simulink model "HIL_Testing_SW"  (Simulink 7.5)
settings: Solver=ode1  StartTime=0.0  StopTime=Inf  FixedStep=0.001  RelTol=1e-3
PostLoadFcn:
  | , if any(exist('dsrtsu_mdlpostloadfcn', 'file') == [2, 3, 6]), try dsrtsu_mdlpostloadfcn('Execute', bdroot); catch fprintf('Error in PostLoadFcn (dsrtsu_mdlpostloadfcn) for model "%s":\n %s\n', bdroot, lasterr); end, end,
undefined symbols (not defined in the file): CeBSER_Cnt_NumTempAxisPts, ChargeCord, ChargeCord_Control, ChargeToSOCCurr, ChrgCurrLim, CrntSens1Fine, CS_SOCSetPt, CyclerMaxChrgPwr, CyclerMaxDschrgPwr, deltaAhr, Drive_1, Drive_10, Drive_11, Drive_12, Drive_13, Drive_14, Drive_15, Drive_16, Drive_17, Drive_18, Drive_19, Drive_2, Drive_20, Drive_21, Drive_22, Drive_23, Drive_24, Drive_25, Drive_26, Drive_27, Drive_28, Drive_29, Drive_3, Drive_30, Drive_31, Drive_32, Drive_33, Drive_34, Drive_35, Drive_36, Drive_37, Drive_38, Drive_39, Drive_4, Drive_40, Drive_41, Drive_42, Drive_43, Drive_44, Drive_45, Drive_46, Drive_47, Drive_48, Drive_49, Drive_5, Drive_50, Drive_51, Drive_6, Drive_7, Drive_8 ... (+50)
libraries: simulink x129, rtican x50, rti2211sailib x5, rti2211serlib x5, rti2202miolib x3
(part 7 of 23)

== system HIL_Testing_SW/LionsHeart/FeaturePresentation/Down_to_Business ==
  CyclerCurrent : Inport  OutDataType=fixdt(1, 16)  OutScaling=2^0
  CyclerVoltage : Inport  Port=2  OutDataType=fixdt(1, 16)  OutScaling=2^0
  BatTemp : Inport  Port=3  OutDataType=fixdt(1, 16)  OutScaling=2^0
  PackVoltage : Inport  Port=4  OutDataType=fixdt(1, 16)  OutScaling=2^0
  PackCurrent : Inport  Port=5  OutDataType=fixdt(1, 16)  OutScaling=2^0
  PackVolt_MaxCell : Inport  Port=6  OutDataType=fixdt(1, 16)  OutScaling=2^0
  PackVolt_MinCell : Inport  Port=7  OutDataType=fixdt(1, 16)  OutScaling=2^0
  Indicator : Inport  Port=8  OutDataType=fixdt(1, 16)  OutScaling=2^0
  CS_SwitchMode : Inport  Port=9  OutDataType=fixdt(1, 16)  OutScaling=2^0
  ESTOP : Inport  Port=10  OutDataType=fixdt(1, 16)  OutScaling=2^0
  ChrgCurrSelect_F : Inport  Port=11  OutDataType=fixdt(1, 16)  OutScaling=2^0
  SOC : Inport  Port=12  OutDataType=fixdt(1, 16)  OutScaling=2^0
  PwrCycle : Inport  Port=13  OutDataType=fixdt(1, 16)  OutScaling=2^0
  Voltage_Cntrl : Inport  Port=14  OutDataType=fixdt(1, 16)  OutScaling=2^0
  Current_Cntrl : Inport  Port=15  OutDataType=fixdt(1, 16)  OutScaling=2^0
  DriveProfile_ModeControl : Subsystem
  Profile_Data : Outport  OutDataType=fixdt(1, 16)  OutScaling=2^0
  CM : Outport  Port=2  OutDataType=fixdt(1, 16)  OutScaling=2^0
  ResetSOC : Outport  Port=3  OutDataType=fixdt(1, 16)  OutScaling=2^0
  VoltTarget : Outport  Port=4  OutDataType=fixdt(1, 16)  OutScaling=2^0
  IndicatorSF : Outport  Port=5  OutDataType=fixdt(1, 16)  OutScaling=2^0
  Profile_Mode : Outport  Port=6  OutDataType=fixdt(1, 16)  OutScaling=2^0
  Script_PwrCycle : Outport  Port=7  OutDataType=fixdt(1, 16)  OutScaling=2^0
  ChargeCurrSelect : Outport  Port=8  OutDataType=fixdt(1, 16)  OutScaling=2^0
  SetChamberT_ToBatTemp : Outport  Port=9  OutDataType=fixdt(1, 16)  OutScaling=2^0
  wires:
  CyclerCurrent/1 -> DriveProfile_ModeControl/1(Current)
  CyclerVoltage/1 -> DriveProfile_ModeControl/2(Voltage)
  BatTemp/1 -> DriveProfile_ModeControl/3(Temp)
  PackVoltage/1 -> DriveProfile_ModeControl/4(PackVoltage)
  PackVolt_MaxCell/1 -> DriveProfile_ModeControl/6(PackVolt_MaxCell)
  PackCurrent/1 -> DriveProfile_ModeControl/5(PackCurrent)
  PackVolt_MinCell/1 -> DriveProfile_ModeControl/7(PackVolt_MinCell)
  Indicator/1 -> DriveProfile_ModeControl/8(Indicator)
  CS_SwitchMode/1 -> DriveProfile_ModeControl/9(CS_ModeSwitch)
  DriveProfile_ModeControl/1(Profile_Data) -> Profile_Data/1
  DriveProfile_ModeControl/2(CM) -> CM/1
  DriveProfile_ModeControl/3(ResetSOC) -> ResetSOC/1
  DriveProfile_ModeControl/4(VoltTarget) -> VoltTarget/1
  DriveProfile_ModeControl/5(IndicatorSF) -> IndicatorSF/1
  DriveProfile_ModeControl/6(Profile_Mode) -> Profile_Mode/1
  ESTOP/1 -> DriveProfile_ModeControl/10(ESTOP)
  ChrgCurrSelect_F/1 -> DriveProfile_ModeControl/11(ChrgCurrSelect_F)
  PwrCycle/1 -> DriveProfile_ModeControl/13(PwrCycle)
  SOC/1 -> DriveProfile_ModeControl/12(SOC)
  DriveProfile_ModeControl/7(Script_PwrCycle) -> Script_PwrCycle/1
  DriveProfile_ModeControl/8(ChargeCurrSelect) -> ChargeCurrSelect/1
  Voltage_Cntrl/1 -> DriveProfile_ModeControl/14(Voltage_Cntrl)
  Current_Cntrl/1 -> DriveProfile_ModeControl/15(Current_Cntrl)
  DriveProfile_ModeControl/9(SetChamberT_ToBatTemp) -> SetChamberT_ToBatTemp/1

== system HIL_Testing_SW/LionsHeart/FeaturePresentation/Safety ==
  BatTemp : Inport  OutDataType=fixdt(1, 16)  OutScaling=2^0
  PackVolt_MinCell : Inport  Port=2  OutDataType=fixdt(1, 16)  OutScaling=2^0
  PackVolt_MaxCell : Inport  Port=3  OutDataType=fixdt(1, 16)  OutScaling=2^0
  Mode : Inport  Port=4  OutDataType=fixdt(1, 16)  OutScaling=2^0
  ContactorStatus : Inport  Port=5  OutDataType=fixdt(1, 16)  OutScaling=2^0
  ChargeMode : Inport  Port=6  OutDataType=fixdt(1, 16)  OutScaling=2^0
  Indicator : Inport  Port=7  OutDataType=fixdt(1, 16)  OutScaling=2^0
  CyclerVoltage : Inport  Port=8  OutDataType=fixdt(1, 16)  OutScaling=2^0
  PackVoltage : Inport  Port=9  OutDataType=fixdt(1, 16)  OutScaling=2^0
  Data Store Read1 : DataStoreRead  DataStoreName=BatTempCold  SampleTime=0
  Data Store Read10 : DataStoreRead  DataStoreName=Voltage_Lid_Cell  SampleTime=0
  Data Store Read11 : DataStoreRead  DataStoreName=MaxCell_Enbl  SampleTime=0
  Data Store Read12 : DataStoreRead  DataStoreName=MinCell_Enbl  SampleTime=0
  Data Store Read13 : DataStoreRead  DataStoreName=UsePackSensor  SampleTime=0
  Data Store Read2 : DataStoreRead  DataStoreName=Voltage_Floor  SampleTime=0
  Data Store Read3 : DataStoreRead  DataStoreName=Voltage_Lid  SampleTime=0
  Data Store Read4 : DataStoreRead  DataStoreName=BatTempHot  SampleTime=0
  Data Store Read5 : DataStoreRead  DataStoreName=FaultTime  SampleTime=0
  Data Store Read6 : DataStoreRead  DataStoreName=Voltage_Floor_Cell  SampleTime=0
  Data Store Read7 : DataStoreRead  DataStoreName=Safety_FloorOffset  SampleTime=0
  Data Store Read8 : DataStoreRead  DataStoreName=Safety_LidOffset  SampleTime=0
  Data Store Read9 : DataStoreRead  DataStoreName=ContactorLine  SampleTime=0
  ResumeFault : Constant  Value=0  OutDataType=fixdt(1, 16)  OutScaling=2^0
  SafetyCheck : Stateflow chart  TreatAsAtomicUnit=on
  Subsystem : Subsystem
  Unit Delay12 : UnitDelay
  fault : DataStoreWrite  DataStoreName=fault  SampleTime=-1
  Control_Mode_Proc : Outport  OutDataType=fixdt(1, 16)  OutScaling=2^0
  wires:
  BatTemp/1 -> SafetyCheck/1(BatTemp)
  PackVolt_MinCell/1 -> SafetyCheck/2(VoltageMin)
  PackVolt_MaxCell/1 -> SafetyCheck/3(VoltageMax)
  Data Store Read4/1 -> SafetyCheck/4(BatTempHot)
  Data Store Read1/1 -> SafetyCheck/5(BatTempCold)
  Data Store Read2/1 -> SafetyCheck/6(Voltage_Floor)
  Data Store Read3/1 -> SafetyCheck/7(Voltage_Lid)
  SafetyCheck/1(Mode_Cntrl) -> Control_Mode_Proc/1
  Indicator/1 -> SafetyCheck/12(SF)
  Unit Delay12/1 -> fault/1
  Data Store Read6/1 -> SafetyCheck/13(Voltage_Floor_Cell)
  Data Store Read10/1 -> SafetyCheck/15(Voltage_Lid_Cell)
  SafetyCheck/2(Fault) -> Unit Delay12/1
  ResumeFault/1 -> SafetyCheck/9(Resume)
  ContactorStatus/1 -> Subsystem/2(ContactorStatus)
  Subsystem/1(CntLine) -> SafetyCheck/10(ContactorLine)
  Subsystem/2(CntStat) -> SafetyCheck/11(ContactorStatus)
  Mode/1 -> SafetyCheck/8(Mode)
  Data Store Read5/1 -> SafetyCheck/16(FaultTime)
  Data Store Read7/1 -> SafetyCheck/17(Safety_FloorOffset)
  Data Store Read8/1 -> SafetyCheck/18(Safety_LidOffset)
  ChargeMode/1 -> Subsystem/3(Chargemode)
  Data Store Read9/1 -> Subsystem/1(ContactorLine)
  PackVoltage/1 -> SafetyCheck/14(VoltagePack)
  CyclerVoltage/1 -> SafetyCheck/19(VoltageCycler)
  Data Store Read11/1 -> SafetyCheck/20(MaxCell_Enbl)
  Data Store Read12/1 -> SafetyCheck/21(MinCell_Enbl)
  Data Store Read13/1 -> SafetyCheck/22(PackSensor)

== system HIL_Testing_SW/LionsHeart/Input Processing/Current Processing ==
  BatteryTemp : Inport  OutDataType=fixdt(1, 16)  OutScaling=2^0
  HVBatCrntLwLmt_CAN : Inport  Port=2  OutDataType=fixdt(1, 16)  OutScaling=2^0
  HVBatCrntUpLmt_CAN : Inport  Port=3  OutDataType=fixdt(1, 16)  OutScaling=2^0
  PackCurrent : Inport  Port=4  OutDataType=fixdt(1, 16)  OutScaling=2^0
  CyclerCurrent : Inport  Port=5  OutDataType=fixdt(1, 16)  OutScaling=2^0
  ChargeTerminationCurrent : Subsystem
  Current Control Select : Subsystem
  CurrentLimit_Charge : Subsystem
  CurrentLimit_Discharge : Subsystem
  Current_Cntrl : Outport  OutDataType=fixdt(1, 16)  OutScaling=2^0
  wires:
  BatteryTemp/1 -> [BatTemp]
  [BatTemp] -> CurrentLimit_Discharge/1(BatteryTemp)
  [BatTemp] -> CurrentLimit_Charge/1(BatteryTemp)
  [BatTemp] -> ChargeTerminationCurrent/1(BatteryTemp)
  HVBatCrntLwLmt_CAN/1 -> CurrentLimit_Discharge/2(HVBatCrntLwLmt_CAN)
  HVBatCrntUpLmt_CAN/1 -> CurrentLimit_Charge/2(HVBatCrntUpLmt_CAN)
  PackCurrent/1 -> Current Control Select/1(PackCurrent)
  CyclerCurrent/1 -> Current Control Select/2(CyclerCurrent)
  Current Control Select/1(Current_Cntrl) -> Current_Cntrl/1

== system HIL_Testing_SW/LionsHeart/Input Processing/Power ==
  CyclerCurrent : Inport  OutDataType=fixdt(1, 16)  OutScaling=2^0
  CyclerVoltage : Inport  Port=2  OutDataType=fixdt(1, 16)  OutScaling=2^0
  Constant : Constant  Value=1000  OutDataType=sfix(16)  OutScaling=2^0
  Divide : Product  Inputs=*/  OutDataType=sfix(16)  OutScaling=2^-10
  Product : Product  OutDataType=sfix(16)  OutScaling=2^0  RndMeth=Zero
  Terminator : Terminator
  wires:
  Constant/1 -> Divide/2
  Product/1 -> Divide/1
  Divide/1 -> Terminator/1  "Power"
  CyclerCurrent/1 -> Product/1
  CyclerVoltage/1 -> Product/2

== system HIL_Testing_SW/LionsHeart/Input Processing/Time ==
  Timestamp_A : Inport  OutDataType=fixdt(1, 16)  OutScaling=2^0
  Data Store Write23 : DataStoreWrite  DataStoreName=StartTimestamp  SampleTime=-1
  Data Store Write24 : DataStoreWrite  DataStoreName=TimeRunning  SampleTime=-1
  Detect Rise Positive : simulink/Logic and Bit Operations/Detect Rise Positive  SystemSampleTime=-1  vinit=0
  DetermineStartTimestamp : Subsystem  TreatAsAtomicUnit=on
  DetermineTimeRunning : Subsystem  TreatAsAtomicUnit=on
  Gain : Gain  ParameterDataType=sfix(16)  ParameterScaling=2^0  OutDataType=sfix(16)  OutScaling=2^0  OutDataTypeStr=Inherit: Same as input
  GetStartTimestamp : DataStoreRead  DataStoreName=StartTimestamp  SampleTime=0
  GetStartTimestamp1 : DataStoreRead  DataStoreName=RUN_TEST  SampleTime=0
  Unit Delay : UnitDelay  SampleTime=-1
  wires:
  Detect Rise Positive/1 -> DetermineStartTimestamp/Enable
  Timestamp_A/1 -> DetermineStartTimestamp/1(Timestamp_A), DetermineTimeRunning/1(Timestamp_A)
  DetermineStartTimestamp/1(StartTimestamp) -> Data Store Write23/1
  GetStartTimestamp/1 -> DetermineTimeRunning/2(StartTimestamp)
  DetermineTimeRunning/1(TimeRunning) -> Data Store Write24/1
  Unit Delay/1 -> DetermineTimeRunning/Enable
  Gain/1 -> Unit Delay/1
  GetStartTimestamp1/1 -> Gain/1, Detect Rise Positive/1

== system HIL_Testing_SW/LionsHeart/Input Processing/Voltage Processing ==
  MinCell : Inport  OutDataType=fixdt(1, 16)  OutScaling=2^0
  MaxCell : Inport  Port=2  OutDataType=fixdt(1, 16)  OutScaling=2^0
  BatteryTemp : Inport  Port=3  OutDataType=fixdt(1, 16)  OutScaling=2^0
  MinSectionVoltage_EREV : Inport  Port=4  OutDataType=fixdt(1, 16)  OutScaling=2^0
  VoltageTarget : Inport  Port=5  OutDataType=fixdt(1, 16)  OutScaling=2^0
  PackVoltage : Inport  Port=6  OutDataType=fixdt(1, 16)  OutScaling=2^0
  HVBatVltLwLmt_CAN : Inport  Port=7  OutDataType=fixdt(1, 16)  OutScaling=2^0
  HVBatVltUpLmt_CAN : Inport  Port=8  OutDataType=fixdt(1, 16)  OutScaling=2^0
  CyclerVoltage : Inport  Port=9  OutDataType=fixdt(1, 16)  OutScaling=2^0
  ChargeTermVoltage : Subsystem
  MaxCell_System : Subsystem
  MinCell_System : Subsystem
  PackVLid : Subsystem
  PackVfloor : Subsystem
  Voltage Control Select : Subsystem
  PackVolt_MinCell : Outport  OutDataType=fixdt(1, 16)  OutScaling=2^0
  PackVolt_MaxCell : Outport  Port=2  OutDataType=fixdt(1, 16)  OutScaling=2^0
  Voltage_Cntrl : Outport  Port=3  OutDataType=fixdt(1, 16)  OutScaling=2^0
  wires:
  MinCell_System/1(PackVolt_MinCell) -> PackVolt_MinCell/1, [MinCellPackEquiv]
  MaxCell_System/1(PackVolt_MaxCell) -> PackVolt_MaxCell/1, [MaxCellPackEquiv]
  BatteryTemp/1 -> [BatTemp]
  [BatTemp] -> PackVLid/2(BatteryTemp)
  [BatTemp] -> PackVfloor/2(BatteryTemp)
  [BatTemp] -> ChargeTermVoltage/1(BatteryTemp)
  VoltageTarget/1 -> ChargeTermVoltage/2(VoltageTarget)
  MinSectionVoltage_EREV/1 -> [MinSectionVoltage_EREV]
  [MinSectionVoltage_EREV] -> PackVfloor/3(MinSectionVoltage)
  PackVoltage/1 -> [PackVoltage]
  [PackVoltage] -> PackVfloor/1(PackVoltage)
  [MinCellPackEquiv] -> PackVfloor/4(MinCellPackEquiv)
  [PackVoltage] -> PackVLid/1(PackVoltage)
  [MaxCellPackEquiv] -> PackVLid/3(MaxCellPackEquiv)
  MinCell/1 -> MinCell_System/1(MinCell)
  MaxCell/1 -> MaxCell_System/1(MaxCell)
  HVBatVltLwLmt_CAN/1 -> PackVfloor/5(HVBatVltLwLmt_CAN)
  HVBatVltUpLmt_CAN/1 -> PackVLid/4(HVBatVltUpLmt_CAN)
  CyclerVoltage/1 -> Voltage Control Select/2(CyclerVoltage)
  [PackVoltage] -> Voltage Control Select/1(PackVoltage)
  Voltage Control Select/1(Voltage_Cntrl) -> Voltage_Cntrl/1

== system HIL_Testing_SW/LionsHeart/OutputProcessing/Apply_BSE_PowerLimits ==
  ControlValue : Inport  OutDataType=sfix(16)  OutScaling=2^0
  LT_PwrDschLmt : Inport  Port=2  OutDataType=sfix(16)  OutScaling=2^0
  SwitchPowerLimit : Inport  Port=3  OutDataType=sfix(16)  OutScaling=2^0
  LT_PwrChgLmt : Inport  Port=4  OutDataType=sfix(16)  OutScaling=2^0
  ControlMode : Inport  Port=5  OutDataType=sfix(16)  OutScaling=2^0
  Compare To Constant : simulink/Logic and Bit Operations/Compare To Constant  SystemSampleTime=-1  relop===  const=2  LogicOutDataTypeMode=uint8  ZeroCross=off
  Constant1 : Constant  Value=1000  OutDataType=sfix(16)  OutScaling=2^0
  Constant2 : Constant  Value=-1000  OutDataType=sfix(16)  OutScaling=2^0
  Current_Cntrl : Constant  Value=0.05/0.04  OutDataType=sfix(16)  OutScaling=2^0
  Multiport Switch : MultiPortSwitch  DataPortOrder=Zero-based contiguous  Inputs=4  zeroidx=on  OutDataType=sfix(16)  OutScaling=2^0
  Power_Cntrl : Constant  Value=0.05/10  OutDataType=sfix(16)  OutScaling=2^0
  Product : Product  OutDataType=sfix(16)  OutScaling=2^0  RndMeth=Zero
  Product1 : Product  OutDataType=sfix(16)  OutScaling=2^0  RndMeth=Zero
  Product2 : Product  OutDataType=sfix(16)  OutScaling=2^0  RndMeth=Zero
  Saturation : Saturate  UpperLimit=-1000  LowerLimit=-200000  OutDataType=sfix(16)  OutScaling=2^0
  Saturation Dynamic : simulink/Discontinuities/Saturation Dynamic  SystemSampleTime=-1  OutMin=[]  OutMax=[]  OutDataTypeStr=Inherit: Same as second input  OutDataType=sfix(16)  OutScaling=2^-10  DoSatur=off
  Standby : Constant  OutDataType=sfix(16)  OutScaling=2^0
  Switch : Switch  Threshold=.5  OutDataType=sfix(16)  OutScaling=2^0
  Switch2 : Switch  Threshold=.5  OutDataType=sfix(16)  OutScaling=2^0
  Voltage_Cntrl : Constant  OutDataType=sfix(16)  OutScaling=2^0
  Control_Value_Proc : Outport  OutDataType=fixdt(1, 16)  OutScaling=2^0
  wires:
  ControlValue/1 -> [Raw_Value]
  ControlMode/1 -> [Mode]
  [Mode] -> Multiport Switch/1
  Voltage_Cntrl/1 -> Multiport Switch/2
  Current_Cntrl/1 -> Multiport Switch/3
  Power_Cntrl/1 -> Multiport Switch/4
  Standby/1 -> Multiport Switch/5
  Multiport Switch/1 -> Product/1
  [Raw_ValueProc] -> Product/2
  Product/1 -> Control_Value_Proc/1
  SwitchPowerLimit/1 -> Switch/2
  LT_PwrDschLmt/1 -> Product1/1
  Constant2/1 -> Product1/2
  Constant1/1 -> Product2/2
  LT_PwrChgLmt/1 -> Product2/1
  [Mode] -> Compare To Constant/1
  Compare To Constant/1 -> Switch2/2
  Switch/1 -> Switch2/1
  [Raw_Value] -> Switch2/3
  [Raw_Value] -> Switch/1
  Switch2/1 -> [Raw_ValueProc]
  [Raw_Value] -> Saturation Dynamic/2
  Product2/1 -> Saturation Dynamic/1
  Saturation Dynamic/1 -> Switch/3
  Product1/1 -> Saturation/1
  Saturation/1 -> Saturation Dynamic/3

== system HIL_Testing_SW/RTI Data/RTI Data Store/RTI Data Store ==
  RTI Data Store : Subsystem
      mask Type: RTI_DATA_STORE
      mask Description:
      | RTI Data Store Block. This block is used by RTI to store internal model dependent data. Deleting this block will result in data loss.
      | 
      | NEVER DELETE, COPY, OR MODIFY THIS BLOCK!
      mask Help:
      | RTI Data Store Block. This block is used by RTI to store internal model dependent data. Deleting this block will result in data loss.
      | 
      | NEVER DELETE, COPY, OR MODIFY THIS BLOCK!
      mask Display: text(0.5, 0.5, ' ', 'HorizontalAlignment', 'center');

== system HIL_Testing_SW/RX/Read BAS3/PID_Reads ==
  Enable : EnablePort
  BatTempSub : Subsystem
  Chart : Stateflow chart  TreatAsAtomicUnit=on
  Fcn : Fcn  Expr=256*u(2)+u(1)
  MaxCellSub : Subsystem
  MinCellSub : Subsystem
  Mux : Mux  Inputs=2
  Mux1 : Mux  Inputs=2
  Relational Operator : RelationalOperator  Operator===  LogicOutDataTypeMode=boolean  LogicDataType=fixdt(0, 8)  OutDataTypeStr=boolean
  Relational Operator1 : RelationalOperator  Operator===  LogicOutDataTypeMode=boolean  LogicDataType=fixdt(0, 8)  OutDataTypeStr=boolean
  Relational Operator2 : RelationalOperator  Operator===  LogicOutDataTypeMode=boolean  LogicDataType=fixdt(0, 8)  OutDataTypeStr=boolean
  Subsystem : Subsystem
  Terminator_{5..8,10..16} (11 alike) : Terminator
  Transmit1 : Constant  Value=17195  OutDataType=fixdt(1, 16)  OutScaling=2^0  OutDataTypeStr=Inherit: Inherit via back propagation
  Transmit2 : Constant  Value=17231  OutDataType=fixdt(1, 16)  OutScaling=2^0  OutDataTypeStr=Inherit: Inherit via back propagation
  Transmit5 : Constant  Value=0.025  OutDataType=fixdt(1, 16)  OutScaling=2^0  OutDataTypeStr=Inherit: Inherit via back propagation
  Transmit9 : Constant  Value=17193  OutDataType=fixdt(1, 16)  OutScaling=2^0  OutDataTypeStr=Inherit: Inherit via back propagation
  USDT_Req_to_VICM_HS : rtican/RTICAN Receive (RX)   SystemSampleTime=-1  Reserved1=[]  Reserved2=[]  Reserved3=[]  Reserved4=[]  SfcnMessage=[]  Msg_Struct=[]  BoardTypeNo=[]  BoardNo=[]  ChannelNo=[]  Parameters=[]  DialogFcn=[]  UnitName=[]  Revision=[]  UnitValues=[]  DSProperties=struct('RTI',struct('Version',uint32(5),'BlockType',struct('isSLSource',uint8(1),'isSLSink',uint8(1),'isHWSource',uint8(0),'isHWSink',uint8(0),'isSetup',uint8(0),'isInline',uint8(1),'isNonInline',uint8(0),'isInterrupt',uint8(0),'isChannelwise',uint8(0)),'IOBoardType','RTICAN','UnitType','MESSAGE','Identifier','RX','DialogType','MSVC','BlockSet','RTICAN','SlaveProcessor','CAN'))  RTIBlockInterface=struct('OutputPortsWidth',int32([1 1 1 1 1 1 1 1 1 1 1]),'OutputPortsActive',[1 1 1 1 1 1 1 1 1 1 1],'OutputPortsName',{{'DgnInf_1','DgnInf_2','DgnInf_3','DgnInf_4','DgnInf_5','DgnInf_6','DgnInf_7','DgnInf_8',['RX status'],['RX time'],['RX delta time']}},'OutputPortsDataType',{{'SS_DOUBLE','SS_DOUBLE','SS_DOUBLE','SS_DOUBLE','SS_DOUBLE','SS_DOUBLE','SS_DOUBLE','SS_DOUBLE','SS_DOUBLE','SS_DOUBLE','SS_DOUBLE'}},'OutputPortsLabel',{{'DgnInf_1','DgnInf_2','DgnInf_3','DgnInf_4','DgnInf_5','DgnInf_6','DgnInf_7','DgnInf_8','','',''}},'OutputPortsLabelMode','ON','InputPortsWidth',int32(0),'InputPortsActive',0,'DialogFcn','rtican_message_interface_gui','BlockDisplay',{{'','center'}},'IconTransparency','on','ParameterTunableNames',{{}},'InitLevel',3,'BlockName',struct('Token',{{'USDT_Req_to_VICM_HS'}}),'SampleTime',{{-1}},'TriggerPort',{{'none'}},'EnablePort',{{'none'}})  RTIBlockParameters=struct('BoardTypeNo',{{4302,'OFF',[]}},'BoardNo',{{1,'ON',[1 16]}},'ChannelNo',{{1,'ON',[1 4]}},'Parameters',{{struct('DataFileSupport',struct('DataFileSelectedMaster',1,'DataFileSelectedLocal',1,'DataFileName',['c:\data\databases\6.4.1\globala - hs.dbc|'],'DataFileDate',['24-Apr-2014 15:37:04'],'SelectedFile',['..\databases\8.4.5 (140425)\globala - hs.dbc'],'InterfaceFcn','rtican_dbc_file_parser'),'Options',struct('StatusSelected',1,'TimeSelected',1,'DeltaTimeSelected',1,'BytePortSelected',0,'MessageLengthSelected',0,'TriggerPort',struct('Selected',0,'TriggerType',0),'UserCoding',struct('Selected',0,'InterfaceFile','UserDecodingFile','FcnName','UserDecodeFcn','InportSelected',0,'InportWidth',1,'OutportSelected',0,'OutportWidth',1),'EnablePortSelected',0,'SignalOnPortnameSelected',1,'UseRXService',0),'Message',struct('MsgOnBlocknameSelected',1,'MsgName','USDT_Req_to_VICM_HS','MsgIdFormat',0,'MsgId',2020,'MsgLength',8,'NumSignals',8,'SampleTime',-1,'Signal',struct('SgnName',{'DgnInf_1','DgnInf_2','DgnInf_3','DgnInf_4','DgnInf_5','DgnInf_6','DgnInf_7','DgnInf_8'},'SgnStartBit',{0,8,16,24,32,40,48,56},'SgnLength',{8,8,8,8,8,8,8,8},'ByteLayout',{2,2,2,2,2,2,2,2},'Factor',{1,1,1,1,1,1,1,1},'Offset',{0,0,0,0,0,0,0,0},'SgnComment',{'','','','','','','',''},'SgnUnit',{'byte','byte','byte','byte','byte','byte','byte','byte'},'Min',{0,0,0,0,0,0,0,0},'Max',{255,255,255,255,255,255,255,255},'SgnType',{0,0,0,0,0,0,0,0},'SLDataType',{'SS_DOUBLE','SS_DOUBLE','SS_DOUBLE','SS_DOUBLE','SS_DOUBLE','SS_DOUBLE','SS_DOUBLE','SS_DOUBLE'},'DataType',{0,0,0,0,0,0,0,0},'ModeValue',{-1,-1,-1,-1,-1,-1,-1,-1}),'MsgIdNumFormat',0,'MsgComment',{{''}}),'Version',1.2,'general',struct('isFromLib',0)),'OFF',[]}},'GroupId',{{struct('Group',{{'RTICAN'}},'No',8,'Behavior',{{'NAMECHANGE'}},'BlockType',{{'SINK'}},'NameChangeFlag',0),'OFF',[]}},'SFcnRTICANMessage',{{struct('MsgType','RX','SFcnPortType','Scalar','MsgName','USDT_Req_to_VICM_HS','MsgIdFormat','STD','MsgId',2020,'MsgLength',8,'NumSignals',8,'SampleTime',-1,'Signal',struct('SgnName',{'DgnInf_1','DgnInf_2','DgnInf_3','DgnInf_4','DgnInf_5','DgnInf_6','DgnInf_7','DgnInf_8'},'SgnStartBit',{0,8,16,24,32,40,48,56},'SgnLength',{8,8,8,8,8,8,8,8},'ByteLayout',{['motorola back.'],['motorola back.'],['motorola back.'],['motorola back.'],['motorola back.'],['motorola back.'],['motorola back.'],['motorola back.']},'Factor',{1,1,1,1,1,1,1,1},'Offset',{0,0,0,0,0,0,0,0},'SgnType',{'standard','standard','standard','standard','standard','standard','standard','standard'},'SLDataType',{'SS_DOUBLE','SS_DOUBLE','SS_DOUBLE','SS_DOUBLE','SS_DOUBLE','SS_DOUBLE','SS_DOUBLE','SS_DOUBLE'},'DataType',{['unsigned int'],['unsigned int'],['unsigned int'],['unsigned int'],['unsigned int'],['unsigned int'],['unsigned int'],['unsigned int']},'ModeValue',{-1,-1,-1,-1,-1,-1,-1,-1}),'StatusSelected','yes','TimeSelected','yes','DeltaTimeSelected','yes','BytePortSelected','no','MessageLengthSelected','no','TriggerPort',struct('Selected','no','TriggerType',0),'UserCoding',struct('Selected','no','InterfaceFile','UserDecodingFile','FcnName','UserDecodeFcn','InportSelected','no','InportWidth',1,'OutportSelected','no','OutportWidth',1),'EnablePortSelected','no','UseRXService','no','BoardType','DS4302','BoardNo',1,'ControllerNo',1),'OFF',[]}},'TLCFileName',{{'rtican_rx_message','OFF',[]}})  RTISFcnParameters=struct('SFcnRTICANMessage','struct','TLCFileName','char')  RTIBlockParaDefault=struct('BoardTypeNo',4302,'BoardNo',1,'ChannelNo',1,'Parameters',struct('DataFileSupport',struct('DataFileSelectedMaster',0,'DataFileSelectedLocal',0,'DataFileName','','DataFileDate','','SelectedFile',['<no file selected>']),'Options',struct('StatusSelected',1,'TimeSelected',1,'DeltaTimeSelected',1,'BytePortSelected',0,'MessageLengthSelected',0,'TriggerPort',struct('Selected',0,'TriggerType','rising'),'UserCoding',struct('Selected',0,'InterfaceFile','UserDecodingFile','FcnName','UserDecodeFcn','InportSelected',0,'InportWidth',1,'OutportSelected',0,'OutportWidth',1),'EnablePortSelected',0,'SignalOnPortnameSelected',1,'UseRXService',0),'Message',struct('MsgOnBlocknameSelected',0,'MsgName',['RX Message'],'MsgIdFormat',0,'MsgId',100,'MsgLength',8,'NumSignals',1,'SampleTime',-1,'Signal',struct('SgnName',['RX signal'],'SgnStartBit',0,'SgnLength',8,'SgnType',0,'ModeValue',-1,'DataType',0,'SLDataType','SS_DOUBLE','ByteLayout',0,'Factor',1,'Offset',0,'Min',0,'Max',255,'SgnComment',{{}},'SgnUnit',''),'MsgIdNumFormat',0,'MsgComment',{{''}}),'Version',1.2,'general',struct('isFromLib',1)),'GroupId',struct('Group',{{'RTICAN'}},'No',1,'Behavior',{{'NAMECHANGE'}},'BlockType',{{'SINK'}},'NameChangeFlag',0),'SFcnRTICANMessage',struct('MsgType','RX','MsgName',['RX Message'],'MsgIdFormat','STD','MsgId',100,'MsgLength',8,'NumSignals',1,'SampleTime',-1,'Signal',struct('SgnName',['RX signal'],'SgnStartBit',0,'SgnLength',8,'SgnType','standard','ModeValue',-1,'DataType',['unsigned int'],'ByteLayout',['little endian'],'SLDataType','SS_DOUBLE','Factor',1,'Offset',0),'StatusSelected','yes','TimeSelected','yes','DeltaTimeSelected','yes','BytePortSelected','no','MessageLengthSelected','no','EnablePortSelected','no','UserCoding',struct('Selected','no','InterfaceFile','UserDecodingFile','FcnName','UserDecodeFcn','InportSelected','no','InportWidth',1,'OutportSelected','no','OutportWidth',1),'TriggerPort',struct('Selected','no','TriggerType','rising'),'UseRXService','no','BoardType','DS4302','BoardNo',1,'ControllerNo',1,'SFcnPortType','Scalar'),'TLCFileName','rtican_rx_message')
      settings: AttributesFormatString=Group Id: RTICAN8\n
  USDT_Req_to_VICM_HS1 : rtican/RTICAN Transmit (TX)   SystemSampleTime=-1  Reserved1=[]  Reserved2=[]  Reserved3=[]  Reserved4=[]  SfcnMessage=[]  Msg_Struct=[]  BoardTypeNo=[]  BoardNo=[]  ChannelNo=[]  Parameters=[]  DialogFcn=[]  UnitName=[]  Revision=[]  UnitValues=[]  DSProperties=struct('RTI',struct('Version',uint32(5),'BlockType',struct('isSLSource',uint8(1),'isSLSink',uint8(1),'isHWSource',uint8(0),'isHWSink',uint8(0),'isSetup',uint8(0),'isInline',uint8(1),'isNonInline',uint8(0),'isInterrupt',uint8(0),'isChannelwise',uint8(0)),'IOBoardType','RTICAN','UnitType','MESSAGE','Identifier','TX','DialogType','MSVC','BlockSet','RTICAN','SlaveProcessor','CAN'))  RTIBlockInterface=struct('InputPortsWidth',int32([1 1 1 1 1 1 1 1]),'InputPortsActive',[1 1 1 1 1 1 1 1],'InputPortsName',{{'DgnInf_1','DgnInf_2','DgnInf_3','DgnInf_4','DgnInf_5','DgnInf_6','DgnInf_7','DgnInf_8'}},'InputPortsDataType',{{'SS_DOUBLE','SS_DOUBLE','SS_DOUBLE','SS_DOUBLE','SS_DOUBLE','SS_DOUBLE','SS_DOUBLE','SS_DOUBLE'}},'OutputPortsWidth',int32([1 1 1 1]),'OutputPortsActive',[1 1 1 1],'OutputPortsName',{{['TX status'],['TX time'],['TX delta time'],['TX delay time']}},'DialogFcn','rtican_message_interface_gui','BlockDisplay',{{'','center'}},'IconTransparency','on','InitLevel',3,'BlockName',struct('Token',{{'USDT_Req_to_VICM_HS'}}),'SampleTime',{{-1}},'TriggerPort',{{'none'}},'EnablePort',{{'none'}})  RTIBlockParameters=struct('BoardTypeNo',{{4302,'OFF',[]}},'BoardNo',{{1,'ON',[1 16]}},'ChannelNo',{{1,'ON',[1 4]}},'Parameters',{{struct('DataFileSupport',struct('DataFileSelectedMaster',1,'DataFileSelectedLocal',1,'DataFileName',['c:\data\databases\6.4.1\globala - hs.dbc|'],'DataFileDate',['24-Apr-2014 15:37:04'],'SelectedFile',['..\databases\8.4.5 (140425)\globala - hs.dbc'],'InterfaceFcn','rtican_dbc_file_parser'),'Options',struct('StatusSelected',1,'TimeSelected',1,'DeltaTimeSelected',1,'DelayTimeSelected',1,'DelayTimeTXCommandSelected',0,'EncodeSetUnusedBitsToOne',0,'EnableMsgLoopback',0,'TriggerPort',struct('Selected',0,'TriggerType',0),'EnablePortSelected',0,'SignalOnPortnameSelected',1,'UserCoding',struct('Selected',0,'InterfaceFile','UserEncodingFile','FcnName','UserEncodeFcn','InportSelected',0,'InportWidth',1,'OutportSelected',0,'OutportWidth',1),'TerminationMsg',struct('Selected',0,'Byte0_7','0'),'InitialMsg',struct('Selected',0,'Byte0_7','0')),'Message',struct('MsgOnBlocknameSelected',1,'MsgName','USDT_Req_to_VICM_HS','MsgIdFormat',0,'MsgId',2020,'MsgLength',8,'NumSignals',8,'SampleTime',-1,'StartTime',struct('Selected',0,'Value',0),'AutoRepeatTime',struct('Selected',0,'Value',0.1),'Timeout',struct('Selected',0,'Value',0.1),'DelayTime',struct('Selected',0,'Value',0.1),'Signal',struct('SgnName',{'DgnInf_1','DgnInf_2','DgnInf_3','DgnInf_4','DgnInf_5','DgnInf_6','DgnInf_7','DgnInf_8'},'SgnStartBit',{0,8,16,24,32,40,48,56},'SgnLength',{8,8,8,8,8,8,8,8},'ByteLayout',{2,2,2,2,2,2,2,2},'Factor',{1,1,1,1,1,1,1,1},'Offset',{0,0,0,0,0,0,0,0},'SgnComment',{'','','','','','','',''},'SgnUnit',{'byte','byte','byte','byte','byte','byte','byte','byte'},'Min',{0,0,0,0,0,0,0,0},'Max',{255,255,255,255,255,255,255,255},'SgnType',{0,0,0,0,0,0,0,0},'SLDataType',{'SS_DOUBLE','SS_DOUBLE','SS_DOUBLE','SS_DOUBLE','SS_DOUBLE','SS_DOUBLE','SS_DOUBLE','SS_DOUBLE'},'DataType',{0,0,0,0,0,0,0,0},'ModeValue',{-1,-1,-1,-1,-1,-1,-1,-1}),'MsgIdNumFormat',0,'MsgComment',{{''}}),'Version',1.2,'general',struct('isFromLib',0)),'OFF',[]}},'GroupId',{{struct('Group',{{'RTICAN'}},'No',8,'Behavior',{{'NAMECHANGE'}},'BlockType',{{'SINK'}},'NameChangeFlag',0),'OFF',[]}},'SFcnRTICANMessage',{{struct('MsgType','TX','SFcnPortType','Scalar','MsgName','USDT_Req_to_VICM_HS','MsgIdFormat','STD','MsgId',2020,'MsgLength',8,'NumSignals',8,'SampleTime',-1,'StartTime',struct('Selected','no','Value',0),'AutoRepeatTime',struct('Selected','no','Value',0.1),'Timeout',struct('Selected','no','Value',0.1),'Signal',struct('SgnName',{'DgnInf_1','DgnInf_2','DgnInf_3','DgnInf_4','DgnInf_5','DgnInf_6','DgnInf_7','DgnInf_8'},'SgnStartBit',{0,8,16,24,32,40,48,56},'SgnLength',{8,8,8,8,8,8,8,8},'ByteLayout',{['motorola back.'],['motorola back.'],['motorola back.'],['motorola back.'],['motorola back.'],['motorola back.'],['motorola back.'],['motorola back.']},'Factor',{1,1,1,1,1,1,1,1},'Offset',{0,0,0,0,0,0,0,0},'SgnType',{'standard','standard','standard','standard','standard','standard','standard','standard'},'SLDataType',{'SS_DOUBLE','SS_DOUBLE','SS_DOUBLE','SS_DOUBLE','SS_DOUBLE','SS_DOUBLE','SS_DOUBLE','SS_DOUBLE'},'DataType',{['unsigned int'],['unsigned int'],['unsigned int'],['unsigned int'],['unsigned int'],['unsigned int'],['unsigned int'],['unsigned int']},'ModeValue',{-1,-1,-1,-1,-1,-1,-1,-1}),'StatusSelected','yes','TimeSelected','yes','DeltaTimeSelected','yes','DelayTimeSelected','yes','DelayTimeTXCommandSelected','no','EncodeSetUnusedBitsToOne','no','EnableMsgLoopback','no','TriggerPort',struct('Selected','no','TriggerType',0),'EnablePortSelected','no','UserCoding',struct('Selected','no','InterfaceFile','UserEncodingFile','FcnName','UserEncodeFcn','InportSelected','no','InportWidth',1,'OutportSelected','no','OutportWidth',1),'TerminationMsg',struct('Selected','no','Byte0','0x00','Byte1','0x00','Byte2','0x00','Byte3','0x00','Byte4','0x00','Byte5','0x00','Byte6','0x00','Byte7','0x00'),'InitialMsg',struct('Selected','no','Byte0','0x00','Byte1','0x00','Byte2','0x00','Byte3','0x00','Byte4','0x00','Byte5','0x00','Byte6','0x00','Byte7','0x00'),'BoardType','DS4302','BoardNo',1,'ControllerNo',1),'OFF',[]}},'TLCFileName',{{'rtican_tx_message','OFF',[]}})  RTISFcnParameters=struct('SFcnRTICANMessage','struct','TLCFileName','char')  RTIBlockParaDefault=struct('BoardTypeNo',4302,'BoardNo',1,'ChannelNo',1,'Parameters',struct('DataFileSupport',struct('DataFileSelectedMaster',0,'DataFileSelectedLocal',0,'DataFileName','','DataFileDate','','SelectedFile',['<no file selected>']),'Options',struct('StatusSelected',1,'TimeSelected',1,'DeltaTimeSelected',1,'DelayTimeSelected',1,'DelayTimeTXCommandSelected',0,'EncodeSetUnusedBitsToOne',0,'EnableMsgLoopback',0,'TriggerPort',struct('Selected',0,'TriggerType','rising'),'EnablePortSelected',0,'SignalOnPortnameSelected',1,'UserCoding',struct('Selected',0,'InterfaceFile','UserEncodingFile','FcnName','UserEncodeFcn','InportSelected',0,'InportWidth',1,'OutportSelected',0,'OutportWidth',1),'TerminationMsg',struct('Selected',0,'Byte0_7','0'),'InitialMsg',struct('Selected',0,'Byte0_7','0')),'Message',struct('MsgOnBlocknameSelected',0,'MsgName',['TX Message'],'MsgIdFormat',0,'MsgId',100,'MsgLength',8,'NumSignals',1,'SampleTime',-1,'StartTime',struct('Selected',0,'Value',0),'AutoRepeatTime',struct('Selected',0,'Value',0.1),'Timeout',struct('Selected',0,'Value',0.1),'DelayTime',struct('Selected',0,'Value',0.1),'Signal',struct('SgnName',['TX signal'],'SgnStartBit',0,'SgnLength',8,'SgnType',0,'ModeValue',-1,'DataType',0,'SLDataType','SS_DOUBLE','ByteLayout',0,'Factor',1,'Offset',0,'Min',0,'Max',255,'SgnComment',{{}},'SgnUnit',''),'MsgIdNumFormat',0,'MsgComment',{{''}}),'Version',1.2,'general',struct('isFromLib',1)),'GroupId',struct('Group',{{'RTICAN'}},'No',1,'Behavior',{{'NAMECHANGE'}},'BlockType',{{'SINK'}},'NameChangeFlag',0),'SFcnRTICANMessage',struct('MsgType','TX','MsgName',['TX Message'],'MsgIdFormat','STD','MsgId',100,'MsgLength',2,'NumSignals',1,'SampleTime',-1,'StartTime',struct('Selected','no','Value',0),'AutoRepeatTime',struct('Selected','no','Value',0.1),'Timeout',struct('Selected','no','Value',0.1),'DelayTime',struct('Selected','no','Value',0.1),'Signal',struct('SgnName',['TX signal'],'SgnStartBit',0,'SgnLength',8,'SgnType','standard','ModeValue',-1,'DataType',['unsigned int'],'ByteLayout',['little endian'],'SLDataType','SS_DOUBLE','Factor',1,'Offset',0),'StatusSelected','yes','TimeSelected','yes','DeltaTimeSelected','yes','DelayTimeSelected','yes','EnablePortSelected','no','EnableMsgLoopback','no','DelayTimeTXCommandSelected','no','EncodeSetUnusedBitsToOne','no','UserCoding',struct('Selected','no','InterfaceFile','UserDecodingFile','FcnName','UserDecodeFcn','InportSelected','no','InportWidth',1,'OutportSelected','no','OutportWidth',1),'TerminationMsg',struct('Selected','no','Byte0','0x00','Byte1','0x00','Byte2','0x00','Byte3','0x00','Byte4','0x00','Byte5','0x00','Byte6','0x00','Byte7','0x00'),'InitialMsg',struct('Selected','no','Byte0','0x00','Byte1','0x00','Byte2','0x00','Byte3','0x00','Byte4','0x00','Byte5','0x00','Byte6','0x00','Byte7','0x00'),'TriggerPort',struct('Selected','no','TriggerType','rising'),'BoardType','DS4302','BoardNo',1,'ControllerNo',1,'SFcnPortType','Scalar'),'TLCFileName','rtican_tx_message')
      settings: AttributesFormatString=Group Id: RTICAN8\n
  MinCell : Outport  OutDataType=fixdt(1, 16)  OutScaling=2^0
  MaxCell : Outport  Port=2  OutDataType=fixdt(1, 16)  OutScaling=2^0
  BatTemp : Outport  Port=3  OutDataType=fixdt(1, 16)  OutScaling=2^0
  wires:
  USDT_Req_to_VICM_HS1/1 -> Terminator_5/1
  USDT_Req_to_VICM_HS1/2 -> Terminator_6/1
  USDT_Req_to_VICM_HS1/3 -> Terminator_7/1
  USDT_Req_to_VICM_HS1/4 -> Terminator_8/1
  Chart/1(Increment) -> [PID_Index]
  [Dgn5] -> USDT_Req_to_VICM_HS1/5
  [Dgn6] -> USDT_Req_to_VICM_HS1/6
  [Dgn7] -> USDT_Req_to_VICM_HS1/7
  [PID] -> Relational Operator/1
  Transmit9/1 -> Relational Operator/2
  Relational Operator/1 -> MinCellSub/Enable
  [Value_raw] -> MinCellSub/1(In)
  [PID_Index] -> Subsystem/1(PID_Index)
  [Dgn1] -> USDT_Req_to_VICM_HS1/1
  [Dgn2] -> USDT_Req_to_VICM_HS1/2
  [Dgn3] -> USDT_Req_to_VICM_HS1/3
  [Dgn4] -> USDT_Req_to_VICM_HS1/4
  Subsystem/1(Dgn8) -> [Dgn8]
  Subsystem/2(Dgn7) -> [Dgn7]
  Subsystem/3(Dgn6) -> [Dgn6]
  Subsystem/4(Dgn5) -> [Dgn5]
  Subsystem/5(Dgn4) -> [Dgn4]
  Subsystem/6(Dgn3) -> [Dgn3]
  Subsystem/7(Dgn2) -> [Dgn2]
  Subsystem/8(Dgn1) -> [Dgn1]
  [PID] -> Relational Operator1/1
  Transmit1/1 -> Relational Operator1/2
  Relational Operator1/1 -> MaxCellSub/Enable
  [Value_raw] -> MaxCellSub/1(In)
  [PID] -> Relational Operator2/1
  Transmit2/1 -> Relational Operator2/2
  Relational Operator2/1 -> BatTempSub/Enable
  [Value_raw] -> BatTempSub/1(In)
  MinCellSub/1(MinCell) -> MinCell/1
  MaxCellSub/1(MaxCell) -> MaxCell/1
  Transmit5/1 -> Chart/1(Timer)
  USDT_Req_to_VICM_HS/6 -> Mux/2  "DgnInf_6"
  USDT_Req_to_VICM_HS/5 -> Mux/1  "DgnInf_5"
  Mux/1 -> [PID_raw]
  [PID_raw] -> Fcn/1
  Fcn/1 -> [PID]
  USDT_Req_to_VICM_HS/4 -> Mux1/2  "DgnInf_4"
  USDT_Req_to_VICM_HS/3 -> Mux1/1  "DgnInf_3"
  Mux1/1 -> [Value_raw]
  USDT_Req_to_VICM_HS/1 -> Terminator_10/1  "DgnInf_1"
  USDT_Req_to_VICM_HS/2 -> Terminator_11/1  "DgnInf_2"
  USDT_Req_to_VICM_HS/7 -> Terminator_12/1  "DgnInf_7"
  USDT_Req_to_VICM_HS/8 -> Terminator_13/1  "DgnInf_8"
  USDT_Req_to_VICM_HS/9 -> Terminator_14/1
  USDT_Req_to_VICM_HS/10 -> Terminator_15/1
  USDT_Req_to_VICM_HS/11 -> Terminator_16/1
  BatTempSub/1(BatTemp) -> BatTemp/1
  [Dgn8] -> USDT_Req_to_VICM_HS1/8
